simulink model "untitled1"  (R2014a)
settings: Solver=ode45  StartTime=0.0  StopTime=0.5  MaxStep=1e-2  RelTol=1e-3  AbsTol=1e-4
undefined symbols (not defined in the file): d_y_com, l0_virtual
libraries: simulink x2
settings Model: Creator=wmartin  LastModifiedBy=wmartin

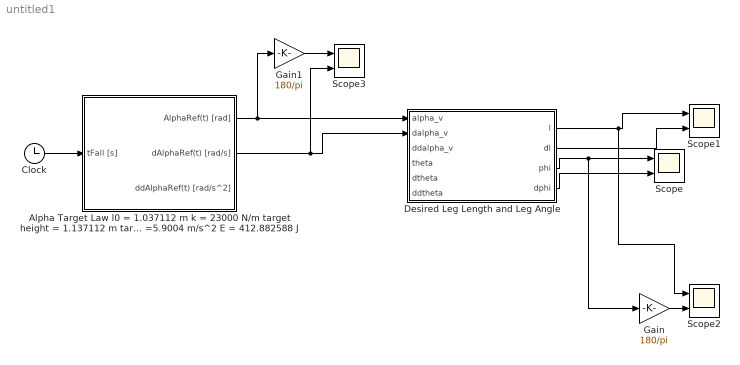
== system untitled1 ==
  Alpha Target Law l0 = 1.037112 m k = 23000 N/m target height = 1.137112 m target speed = 0.5 m/s m = 60.4120 kg g =5.9004 m/s^2 E = 412.882588 J : Subsystem
  Clock : Clock
  Desired Leg Length and Leg Angle : MATLAB Function  TreatAsAtomicUnit=on
  Gain : Gain  Gain=180/pi
  Gain1 : Gain  Gain=180/pi
  Scope{,1..3} (4 alike) : Scope  NumInputPorts=2
      Scope settings: YMin=-5~-5  YMax=5~5
      Scope1 settings: YMin=-5~-5  YMax=5~5
      Scope2 settings: YMin=-5~-5  YMax=5~5  SaveName=ScopeData2
      Scope3 settings: YMin=-5~-5  YMax=5~5  SaveName=ScopeData3
  wires:
  Clock/1 -> Alpha Target Law l0 = 1.037112 m k = 23000 N/m target height = 1.137112 m target speed = 0.5 m/s m = 60.4120 kg g =5.9004 m/s^2 E = 412.882588 J/1(tFall [s])
  Alpha Target Law l0 = 1.037112 m k = 23000 N/m target height = 1.137112 m target speed = 0.5 m/s m = 60.4120 kg g =5.9004 m/s^2 E = 412.882588 J/2(dAlphaRef(t) [rad/s]) -> Scope3/2, Desired Leg Length and Leg Angle/2(dalpha_v)
  Desired Leg Length and Leg Angle/3(phi) -> Gain/1, Scope/1
  Desired Leg Length and Leg Angle/4(dphi) -> Scope/2
  Desired Leg Length and Leg Angle/1(l) -> Scope2/1, Scope1/1
  Desired Leg Length and Leg Angle/2(dl) -> Scope1/2
  Gain/1 -> Scope2/2
  Alpha Target Law l0 = 1.037112 m k = 23000 N/m target height = 1.137112 m target speed = 0.5 m/s m = 60.4120 kg g =5.9004 m/s^2 E = 412.882588 J/1(AlphaRef(t) [rad]) -> Gain1/1, Desired Leg Length and Leg Angle/1(alpha_v)
  Gain1/1 -> Scope3/1

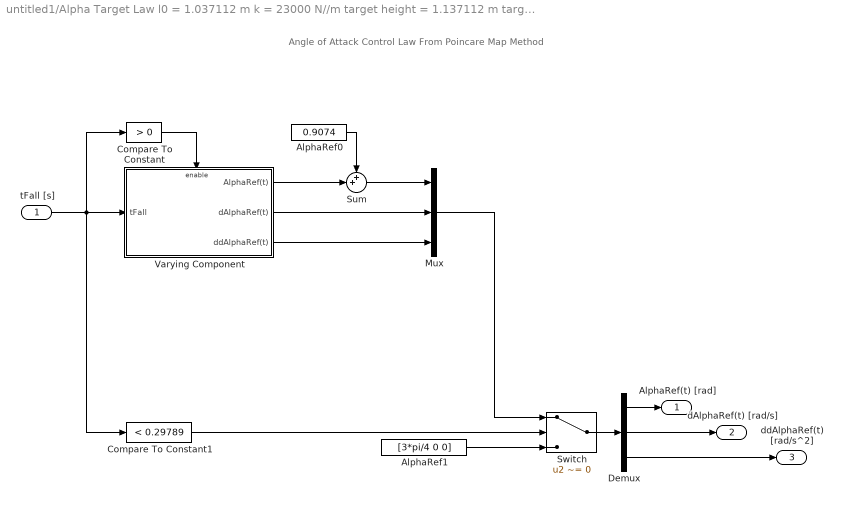
== system untitled1/Alpha Target Law l0 = 1.037112 m k = 23000 N//m target height = 1.137112 m target speed = 0.5 m//s m = 60.4120 kg g =5.9004 m//s^2 E = 412.882588 J ==
  note: Angle of Attack Control Law From Poincare Map Method
  tFall [s] : Inport
  AlphaRef0 : Constant  Value=0.9074
  AlphaRef1 : Constant  Value=[3*pi/4 0 0]
  Compare To Constant : simulink/Logic and Bit Operations/Compare To Constant  relop=>  const=0  OutDataTypeStr=boolean  ZeroCross=off
  Compare To Constant1 : simulink/Logic and Bit Operations/Compare To Constant  relop=<  const=0.29789  OutDataTypeStr=boolean  ZeroCross=off
  Demux : Demux  Outputs=3
  Mux : Mux  Inputs=3
  Sum : Sum  Inputs=++|
  Switch : Switch  Criteria=u2 ~= 0
  Varying Component : Subsystem
  AlphaRef(t) [rad] : Outport
  dAlphaRef(t) [rad/s] : Outport  Port=2
  ddAlphaRef(t) [rad/s^2] : Outport  Port=3
  wires:
  tFall [s]/1 -> Compare To Constant/1, Compare To Constant1/1, Varying Component/1(tFall)
  Varying Component/2(dAlphaRef(t)) -> Mux/2
  Varying Component/3(ddAlphaRef(t)) -> Mux/3
  Compare To Constant/1 -> Varying Component/Enable
  Sum/1 -> Mux/1
  AlphaRef0/1 -> Sum/1
  Compare To Constant1/1 -> Switch/2
  Switch/1 -> Demux/1
  Demux/1 -> AlphaRef(t) [rad]/1
  Demux/2 -> dAlphaRef(t) [rad/s]/1
  Demux/3 -> ddAlphaRef(t) [rad/s^2]/1
  AlphaRef1/1 -> Switch/3
  Varying Component/1(AlphaRef(t)) -> Sum/2
  Mux/1 -> Switch/1

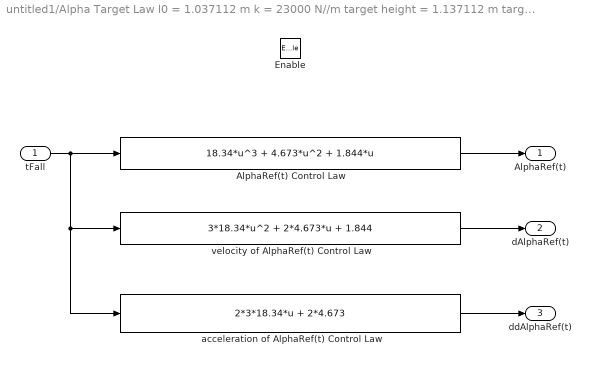
== system untitled1/Alpha Target Law l0 = 1.037112 m k = 23000 N//m target height = 1.137112 m target speed = 0.5 m//s m = 60.4120 kg g =5.9004 m//s^2 E = 412.882588 J/Varying Component ==
  tFall : Inport
  Enable : EnablePort  StatesWhenEnabling=reset  ZeroCross=off
      settings: AttributesFormatString=When enabled: %<StatesWhenEnabling>
  AlphaRef(t) Control Law : Fcn  Expr=18.34*u^3 + 4.673*u^2 + 1.844*u
  acceleration of AlphaRef(t) Control Law : Fcn  Expr=2*3*18.34*u + 2*4.673
  velocity of AlphaRef(t) Control Law : Fcn  Expr=3*18.34*u^2 + 2*4.673*u + 1.844
  AlphaRef(t) : Outport  OutputWhenDisabled=reset  InitialOutput=0
      settings: AttributesFormatString=When disabled: %<OutputWhenDisabled>\nDisabled Output: %<InitialOutput>
  dAlphaRef(t) : Outport  Port=2  OutputWhenDisabled=reset  InitialOutput=0
      settings: AttributesFormatString=When disbaled: %<OutputWhenDisabled>\nDisabled output: %<InitialOutput>
  ddAlphaRef(t) : Outport  Port=3  OutputWhenDisabled=reset  InitialOutput=0
      settings: AttributesFormatString=When disabled: %<OutputWhenDisabled>\nDisabled output: %<InitialOutput>
  wires:
  tFall/1 -> AlphaRef(t) Control Law/1, velocity of AlphaRef(t) Control Law/1, acceleration of AlphaRef(t) Control Law/1
  AlphaRef(t) Control Law/1 -> AlphaRef(t)/1
  velocity of AlphaRef(t) Control Law/1 -> dAlphaRef(t)/1
  acceleration of AlphaRef(t) Control Law/1 -> ddAlphaRef(t)/1

== matlab function untitled1/Desired Leg Length and Leg Angle ==
  data: alpha_v input; dalpha_v input; ddalpha_v input; theta input; dtheta input; ddtheta input; l output; dl output; phi output; d_y_com parameter; l0_virtual parameter; dphi output
function [l, dl, phi, dphi] = fcn(alpha_v, dalpha_v, ddalpha_v, theta, dtheta, ddtheta, d_y_com, l0_virtual)

    l_v = l0_virtual;
    d = d_y_com;
    th = theta;
    dth = dtheta;
    ddth = ddtheta;
    al = alpha_v;
    dal = dalpha_v;
    ddal = ddalpha_v;
    angle = th - al + pi/2;
    
    l = (d^2 + l_v^2 - 2*d*l_v*cos(angle))^0.5;
    phi = pi/2 - th + atan2(l_v*sin(al)-d*cos(th), d*sin(th)+l_v*cos(al));
    if phi < 0, phi = phi + 2*pi; end
    
    dl = 0.5*(d^2 + l_v^2 - 2*d*l_v*cos(angle))^-0.5 * 2*d*l_v*sin(angle)*(dth - dal);
    y_hip = l_v*sin(al)-d*cos(th);
    x_hip = d*sin(th)+l_v*cos(al);
    dphi = -dth + ((x_hip*(l_v*dal*cos(al)+d*dth*sin(th)) - y_hip*(d*dth*cos(th)-l_v*dal*sin(al))) / x_hip^2) / ((y_hip / x_hip)^2 + 1);

end
